simulink model "openloopne"  (R2019b)
settings: Solver=VariableStepAuto  StartTime=0.0  StopTime=400  RelTol=1e-3
InitFcn:
  | L = 0.00056;
  | R = 0.15;
  | ke = 1.3;
  | kt = 0.9725;
  | J = 1;
  | b = 0.1;
settings Model: Creator=srikesh  LastModifiedBy=srikesh

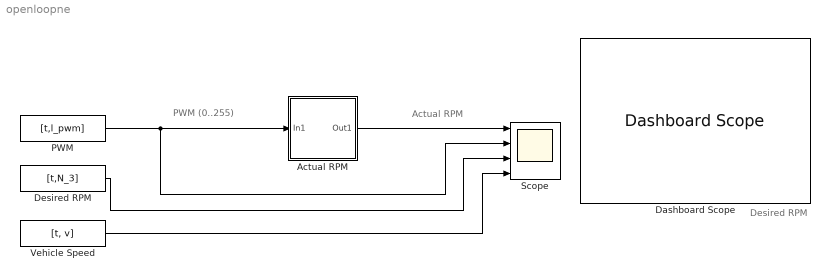
== system openloopne ==
  note: Actual RPM
  note: Desired RPM
  note: PWM (0..255)
  Actual RPM : Subsystem
  Dashboard Scope : DashboardScope
  Desired RPM : FromWorkspace  VariableName=[t,N_3]  SampleTime=0
  PWM : FromWorkspace  VariableName=[t,l_pwm]  SampleTime=0
  Scope : Scope  NumInputPorts=4
  "Vehicle Speed " : FromWorkspace  VariableName=[t, v]  SampleTime=0
  wires:
  "Vehicle Speed "/1 -> Scope/4
  Desired RPM/1 -> Scope/3
  PWM/1 -> Actual RPM/1(In1), Scope/2
  Actual RPM/1(Out1) -> Scope/1

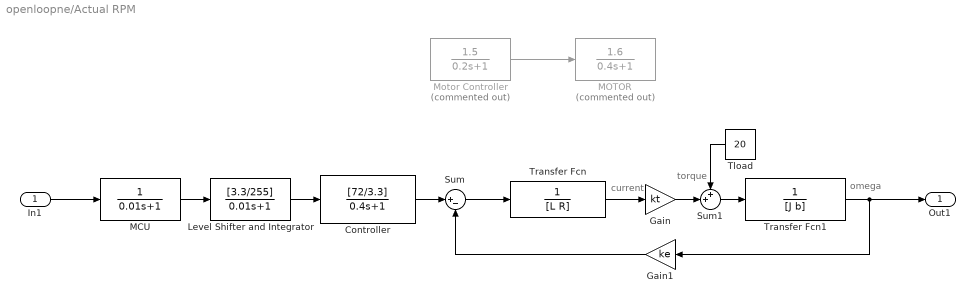
== system openloopne/Actual RPM ==
  note: omega
  note: torque
  note: current
  In1 : Inport
  Controller : TransferFcn  Numerator=[72/3.3]  Denominator=[0.4 1]
  Gain : Gain  Gain=kt
  Gain1 : Gain  Gain=ke
  Level Shifter and Integrator : TransferFcn  Numerator=[3.3/255]  Denominator=[0.01 1]
  MCU : TransferFcn  Denominator=[0.01 1]
  MOTOR : TransferFcn  Commented=on  Numerator=[1.6]  Denominator=[0.4 1]
  Motor Controller : TransferFcn  Commented=on  Numerator=[1.5]  Denominator=[0.2 1]
  Sum : Sum  Inputs=|+-
  Sum1 : Sum  Inputs=++|
  Tload : Constant  Value=20
  Transfer Fcn : TransferFcn  Denominator=[L R]
  Transfer Fcn1 : TransferFcn  Denominator=[J b]
  Out1 : Outport
  wires:
  Motor Controller/1 -> MOTOR/1
  In1/1 -> MCU/1
  MCU/1 -> Level Shifter and Integrator/1
  Transfer Fcn/1 -> Gain/1
  Transfer Fcn1/1 -> Gain1/1, Out1/1
  Gain1/1 -> Sum/2
  Sum/1 -> Transfer Fcn/1
  Sum1/1 -> Transfer Fcn1/1
  Gain/1 -> Sum1/2
  Tload/1 -> Sum1/1
  Level Shifter and Integrator/1 -> Controller/1
  Controller/1 -> Sum/1
